simulink model "Ex_13_Kalman_Estimator"  (Simulink 9.0)
settings: Solver=VariableStepAuto  StartTime=0.0  StopTime=t_max  FixedStep=jointObj.Ts/10  RelTol=1e-3
values from neighbouring files (symbols this model uses):
  t_max = f_max    (= 100)    [Ex_00_example_config.m]
libraries: simulink x1, cjt_library_models x1, cjt_library_observers x1
settings Model: Creator=joern  LastModifiedBy=J�rn
settings DebuggingCC: UnderspecifiedInitializationDetection=Simplified  MergeDetectMultiDrivingBlocksExec=error  SolverPrmCheckMsg=warning
settings GRTTargetCC: GeneratePreprocessorConditionals=Disable all
settings ConfigComp: CovSFcnEnable=off

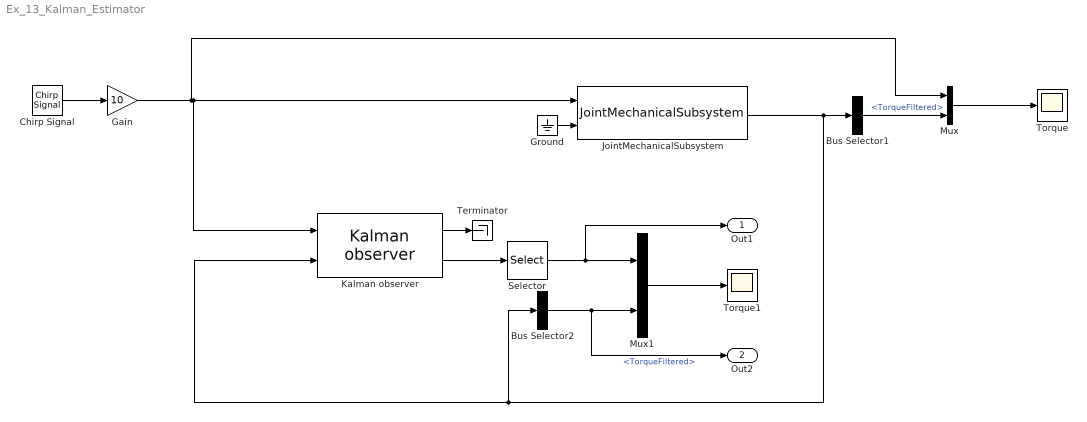
== system Ex_13_Kalman_Estimator ==
  Bus Selector1 : BusSelector  OutputSignals=TorqueFiltered
  Bus Selector2 : BusSelector  OutputSignals=TorqueFiltered
  Chirp Signal : simulink/Sources/Chirp Signal  f1=f_min  T=t_max  f2=f_max
  Gain : Gain  Gain=10
  Ground : Ground
  JointMechanicalSubsystem : cjt_library_models/Joint models/JointMechanicalSubsystem  jointObj=jointObj  fc_vel=1000  fc_torque=1000  input_delay=0  output_delay=1  quantize=on  quantize_bits=19  input_noise_enabled=on  output_noise_enabled=on  var_u=0.12^2  var_y=1.8e-10
  Kalman observer : cjt_library_observers/Observers/Kalman observer  jointObj=My_joint  outputIdx=[2]  var_u=0.12^2  var_y=1.8e-10
  Mux : Mux  Inputs=2
  Mux1 : Mux  Inputs=2
  Selector : Selector  InputPortWidth=7  IndexOptions=Index vector (dialog)  Indices=[7]  OutputSizes=1
  Terminator : Terminator
  Torque : Scope
  Torque1 : Scope
  Out1 : Outport
  Out2 : Outport  Port=2
  wires:
  Mux/1 -> Torque/1
  Ground/1 -> JointMechanicalSubsystem/2
  JointMechanicalSubsystem/1 -> Kalman observer/2, Bus Selector2/1, Bus Selector1/1
  Gain/1 -> Kalman observer/1, JointMechanicalSubsystem/1, Mux/1
  Chirp Signal/1 -> Gain/1
  Bus Selector1/1 -> Mux/2  "<TorqueFiltered>"
  Kalman observer/2 -> Selector/1
  Kalman observer/1 -> Terminator/1
  Bus Selector2/1 -> Out2/1, Mux1/2  "<TorqueFiltered>"
  Selector/1 -> Out1/1, Mux1/1
  Mux1/1 -> Torque1/1
